simulink model "PID_mass_spring_damper_system"  (R2024a)
settings: Solver=ode3  StartTime=0.0  StopTime=inf  FixedStep=0.02  RelTol=1e-3
values from neighbouring files (symbols this model uses):
  b = 2    [param.m]
  k = 0.2    [param.m]
  m = 5    [param.m]
undefined symbols (not defined in the file or in its folder): DiscIntNeverNeededParam
libraries: robotlib x3, slpidlib x1
settings Model: Creator=Aras Güngöre  LastModifiedBy=fp_jin
settings SolverCC: AlgebraicLoopSolver=TrustRegion
settings DebuggingCC: UnconnectedInputMsg=warning  UnconnectedOutputMsg=warning  UnconnectedLineMsg=warning
settings ModelReferenceCC: EnableRefExpFcnMdlSchedulingChecks=on
settings RTWCC: GPUComputeCapability=3.5  DLArmComputeVersion=19.05

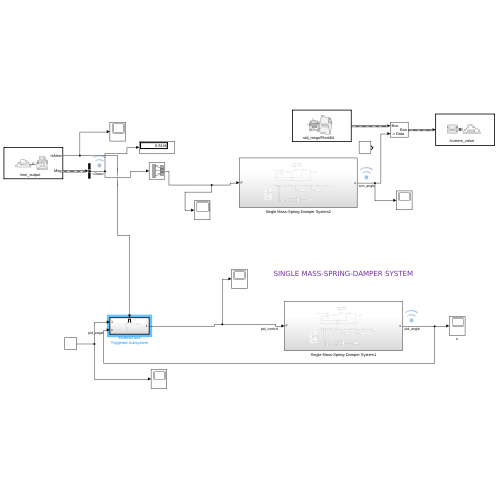
[thumbnail: Simulink's stored preview of the top-level diagram]
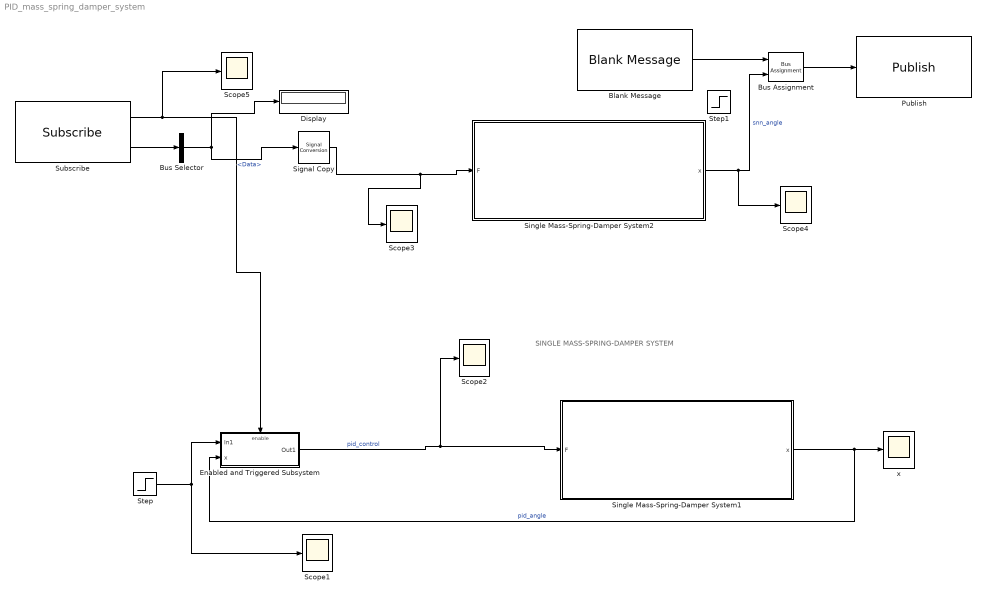
== system PID_mass_spring_damper_system ==
  note: SINGLE MASS-SPRING-DAMPER SYSTEM
  Blank Message : robotlib/Blank Message  messageClass=Message  entityType=std_msgs/Float64  messageType=std_msgs/Float64  SampleTime=-1  legacyBusStruct=off
  Bus Assignment : BusAssignment  AssignedSignals=Data
  Bus Selector : BusSelector  OutputSignals=Data
  Display : Display
  Enabled and Triggered Subsystem : Subsystem  TreatAsAtomicUnit=on
  Publish : robotlib/Publish  topicSource=Specify your own  topic=/current_value  messageType=std_msgs/Float64  legacyBusStruct=off  messageQueueLength=1
  Scope{1..5} (5 alike) : Scope
  Signal Copy : SignalConversion  OverrideOpt=off
  Single Mass-Spring-Damper System1 : Subsystem
  Single Mass-Spring-Damper System2 : Subsystem
  Step : Step  Time=0  After=5
  Step1 : Step  Time=0  After=15  SampleTime=0
  Subscribe : robotlib/Subscribe  topicSource=Specify your own  topic=/snn_output  messageType=std_msgs/Float64  SampleTime=-1  legacyBusStruct=off  messageQueueLength=1
  x : Scope
  wires:
  Blank Message/1 -> Bus Assignment/1
  Bus Assignment/1 -> Publish/1
  Bus Selector/1 -> Display/1, Signal Copy/1  "<Data>"
  Subscribe/2 -> Bus Selector/1
  Step/1 -> Enabled and Triggered Subsystem/1(In1), Scope1/1
  Enabled and Triggered Subsystem/1(Out1) -> Single Mass-Spring-Damper System1/1(F), Scope2/1  "pid_control"
  Single Mass-Spring-Damper System2/1(x) -> Bus Assignment/2, Scope4/1  "snn_angle"
  Signal Copy/1 -> Single Mass-Spring-Damper System2/1(F), Scope3/1
  Subscribe/1 -> Enabled and Triggered Subsystem/Enable, Scope5/1
  Single Mass-Spring-Damper System1/1(x) -> Enabled and Triggered Subsystem/2(x), x/1  "pid_angle"

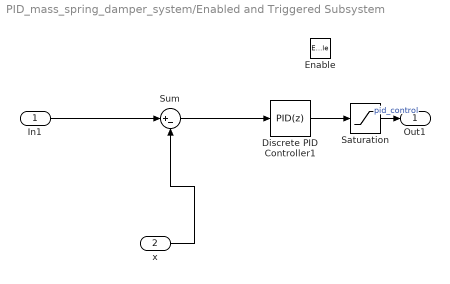
== system PID_mass_spring_damper_system/Enabled and Triggered Subsystem ==
  In1 : Inport
  x : Inport  Port=2
  Enable : EnablePort  StatesWhenEnabling=reset
  Discrete PID Controller1 : slpidlib/PID Controller  Controller=PID  Form=Parallel  TimeDomain=Discrete-time  UseExternalTs=off  SampleTime=-1  IntegratorMethod=Forward Euler  FilterMethod=Forward Euler  ControllerParametersSource=internal  P=1.72  I=0.238*1.0  UseKiTs=off  D=0.2*1.0  UseExternalDerivativeSource=off  N=100  UseFilter=off  TunerSelectOption=Transfer Function Based (PID Tuner App)  InitialConditionSource=internal  InitialConditionForIntegrator=0  InitialConditionForFilter=0  DifferentiatorICPrevScaledInput=0  ExternalReset=none  TrackingMode=off  Kt=1  LimitOutput=off  SatLimitsSource=internal  UpperSaturationLimit=inf  LowerSaturationLimit=-inf  LinearizeAsGain=off  AntiWindupMode=none  Kb=1  LimitIntegrator=off  UpperIntegratorSaturationLimit=inf  LowerIntegratorSaturationLimit=-inf  POutMin=[]  POutMax=[]  IOutMin=[]  IOutMax=[]  DOutMin=[]  DOutMax=[]  NOutMin=[]  NOutMax=[]  SumOutMin=[]  SumOutMax=[]  SaturationOutMin=[]  SaturationOutMax=[]  PParamMin=[]  PParamMax=[]  IParamMin=[]  IParamMax=[]  DParamMin=[]  DParamMax=[]  NParamMin=[]  NParamMax=[]  KbParamMin=[]  KbParamMax=[]  KtParamMin=[]  KtParamMax=[]  KbOutMin=[]  KbOutMax=[]  KtOutMin=[]  KtOutMax=[]  IntegratorOutMin=[]  IntegratorOutMax=[]  FilterOutMin=[]  FilterOutMax=[]  SumI1OutMin=[]  SumI1OutMax=[]  SumI2OutMin=[]  SumI2OutMax=[]  SumI3OutMin=[]  SumI3OutMax=[]  SumI4OutMin=[]  SumI4OutMax=[]  SumDOutMin=[]  SumDOutMax=[]  DifferentiatorOutMin=[]  DifferentiatorOutMax=[]  FilterDiffOutCoefMin=[]  FilterDiffOutCoefMax=[]  ReciprocalOutMin=[]  ReciprocalOutMax=[]  SumDenOutMin=[]  SumDenOutMax=[]  SumNumOutMin=[]  SumNumOutMax=[]  DivideOutMin=[]  DivideOutMax=[]  UdiffTsProdOutMin=[]  UdiffTsProdOutMax=[]  NTsProdOutMin=[]  NTsProdOutMax=[]  UintegralTsProdOutMin=[]  UintegralTsProdOutMax=[]  UngainTsProdOutMin=[]  UngainTsProdOutMax=[]  ClampingZeroOutDataTypeStr=Inherit: Inherit via back propagation  ClampingZeroOutMin=[]  ClampingZeroOutMax=[]  FilterDenConstantOutDataTypeStr=Inherit: Inherit via back propagation  FilterDenConstantOutMin=[]  FilterDenConstantOutMax=[]  PCopyOutDataTypeStr=Inherit: Inherit via back propagation  PCopyOutMin=[]  PCopyOutMax=[]  NCopyOutDataTypeStr=Inherit: Inherit via back propagation  NCopyOutMin=[]  NCopyOutMax=[]  IntegratorContinuousStateAttributes=''  IntegratorStateMustResolveToSignalObject=off  IntegratorRTWStateStorageClass=Auto  FilterContinuousStateAttributes=''  FilterStateMustResolveToSignalObject=off  FilterRTWStateStorageClass=Auto  ParallelPVariant=InternalParameters  IdealPVariant=Disabled  IVariant=InternalParameters  DVariant=InternalParameters  IntegratorVariant=Discrete  SatVariant=Disabled  AWVariant=Passthrough  PCopyVariant=Disabled  TRVariant=Disabled  FdbkBlocksVariant=Forward  IdealPFdbkVariant=Disabled  SatFdbkVariant=Disabled  DerivativeFilterVariant=Differentiator  NVariant=Passthrough  NCopyVariant=Disabled_SignalSpec  FilterICVariant=InternalICsDifferentiator  IntegratorICVariant=InternalICs  ExternalResetVariant=Disabled  TRSumVariant=Passthrough  SumFdbkVariant=Disabled  SumVariant=Sum_PID  TsampFilterVariant=InternalTs  TsampNgainVariant=Passthrough  TsampIntegralVariant=Disabled_SignalSpec  ExternalSaturationOutDataTypeStr=Inherit: Same as second input  DerivativeSourceVariant=ErrorSignal
      settings: LibrarySourceBlock=simulink/Discrete/Discrete PID Controller
  Saturation : Saturate  UpperLimit=20  LowerLimit=-20  LinearizeAsGain=off
  Sum : Sum  Inputs=|+-
  Out1 : Outport
  wires:
  In1/1 -> Sum/1
  Sum/1 -> Discrete PID Controller1/1
  x/1 -> Sum/2
  Discrete PID Controller1/1 -> Saturation/1
  Saturation/1 -> Out1/1  "pid_control"

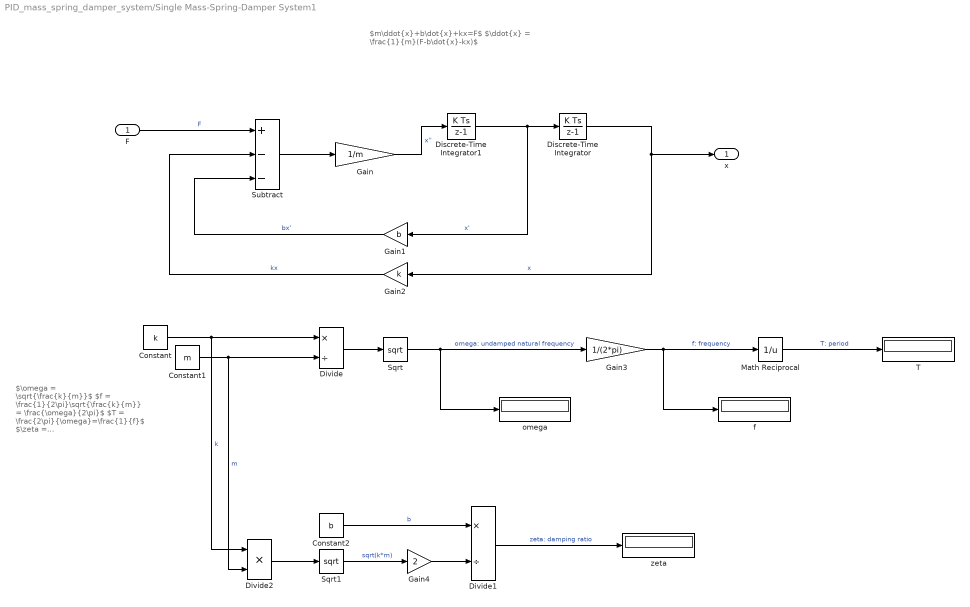
== system PID_mass_spring_damper_system/Single Mass-Spring-Damper System1 ==
  note: $\omega = \sqrt{\frac{k}{m}}$
      | $f = \frac{1}{2\pi}\sqrt{\frac{k}{m}} = \frac{\omega}{2\pi}$
      | $T = \frac{2\pi}{\omega}=\frac{1}{f}$
      | $\zeta = \frac{b}{2\sqrt{km}}$
  note: $m\ddot{x}+b\dot{x}+kx=F$
      | $\ddot{x} = \frac{1}{m}(F-b\dot{x}-kx)$
  F : Inport
  Constant : Constant  Value=k
  Constant1 : Constant  Value=m
  Constant2 : Constant  Value=b
  Discrete-Time Integrator : DiscreteIntegrator  SampleTime=-1  ICPrevOutput=DiscIntNeverNeededParam  ICPrevScaledInput=DiscIntNeverNeededParam
  Discrete-Time Integrator1 : DiscreteIntegrator  SampleTime=-1  ICPrevOutput=DiscIntNeverNeededParam  ICPrevScaledInput=DiscIntNeverNeededParam
  Divide : Product  Inputs=*/
  Divide1 : Product  Inputs=*/
  Divide2 : Product  Inputs=**
  Gain : Gain  Gain=1/m
  Gain1 : Gain  Gain=b
  Gain2 : Gain  Gain=k
  Gain3 : Gain  Gain=1/(2*pi)
  Gain4 : Gain  Gain=2
  Math Reciprocal : Math  Operator=reciprocal  SignedPower=on
  Sqrt : Sqrt
  Sqrt1 : Sqrt
  Subtract : Sum  Inputs=+--
  T : Display
  f : Display
  omega : Display
  zeta : Display
  x : Outport
  wires:
  Gain2/1 -> Subtract/2  "kx"
  Discrete-Time Integrator/1 -> x/1, Gain2/1  "x"
  F/1 -> Subtract/1  "F"
  Gain1/1 -> Subtract/3  "bx'"
  Discrete-Time Integrator1/1 -> Gain1/1, Discrete-Time Integrator/1  "x'"
  Subtract/1 -> Gain/1
  Gain/1 -> Discrete-Time Integrator1/1  "x''"
  Constant/1 -> Divide/1, Divide2/1  "k"
  Constant1/1 -> Divide2/2, Divide/2  "m"
  Divide/1 -> Sqrt/1
  Sqrt/1 -> omega/1, Gain3/1  "omega: undamped natural frequency"
  Gain3/1 -> f/1, Math Reciprocal/1  "f: frequency"
  Math Reciprocal/1 -> T/1  "T: period"
  Constant2/1 -> Divide1/1  "b"
  Sqrt1/1 -> Gain4/1  "sqrt(k*m)"
  Divide2/1 -> Sqrt1/1
  Divide1/1 -> zeta/1  "zeta: damping ratio"
  Gain4/1 -> Divide1/2

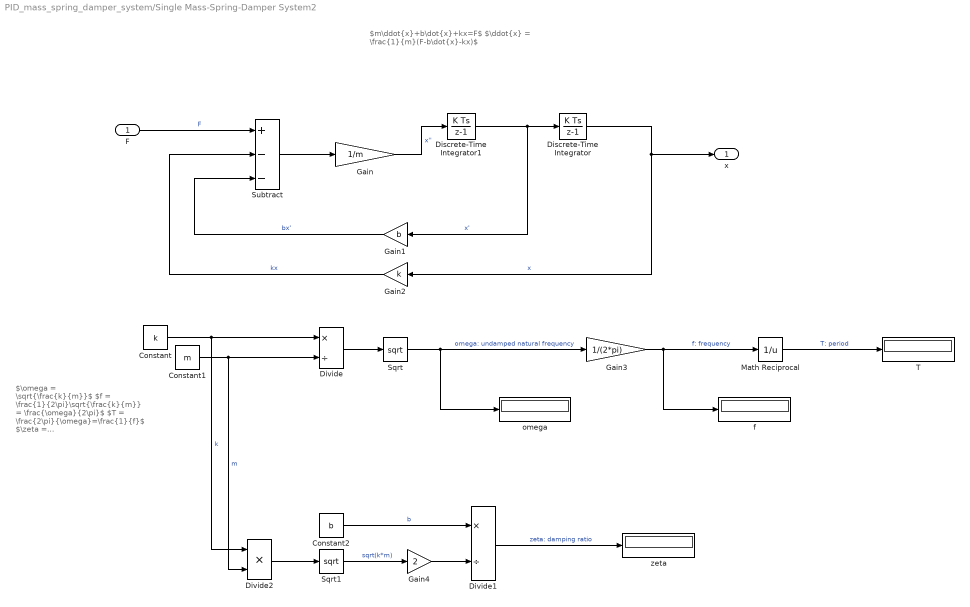
== system PID_mass_spring_damper_system/Single Mass-Spring-Damper System2 ==
  note: $\omega = \sqrt{\frac{k}{m}}$
      | $f = \frac{1}{2\pi}\sqrt{\frac{k}{m}} = \frac{\omega}{2\pi}$
      | $T = \frac{2\pi}{\omega}=\frac{1}{f}$
      | $\zeta = \frac{b}{2\sqrt{km}}$
  note: $m\ddot{x}+b\dot{x}+kx=F$
      | $\ddot{x} = \frac{1}{m}(F-b\dot{x}-kx)$
  F : Inport
  Constant : Constant  Value=k
  Constant1 : Constant  Value=m
  Constant2 : Constant  Value=b
  Discrete-Time Integrator : DiscreteIntegrator  SampleTime=-1  ICPrevOutput=DiscIntNeverNeededParam  ICPrevScaledInput=DiscIntNeverNeededParam
  Discrete-Time Integrator1 : DiscreteIntegrator  SampleTime=-1  ICPrevOutput=DiscIntNeverNeededParam  ICPrevScaledInput=DiscIntNeverNeededParam
  Divide : Product  Inputs=*/
  Divide1 : Product  Inputs=*/
  Divide2 : Product  Inputs=**
  Gain : Gain  Gain=1/m
  Gain1 : Gain  Gain=b
  Gain2 : Gain  Gain=k
  Gain3 : Gain  Gain=1/(2*pi)
  Gain4 : Gain  Gain=2
  Math Reciprocal : Math  Operator=reciprocal  SignedPower=on
  Sqrt : Sqrt
  Sqrt1 : Sqrt
  Subtract : Sum  Inputs=+--
  T : Display
  f : Display
  omega : Display
  zeta : Display
  x : Outport
  wires:
  Gain2/1 -> Subtract/2  "kx"
  Discrete-Time Integrator/1 -> x/1, Gain2/1  "x"
  F/1 -> Subtract/1  "F"
  Gain1/1 -> Subtract/3  "bx'"
  Discrete-Time Integrator1/1 -> Gain1/1, Discrete-Time Integrator/1  "x'"
  Subtract/1 -> Gain/1
  Gain/1 -> Discrete-Time Integrator1/1  "x''"
  Constant/1 -> Divide/1, Divide2/1  "k"
  Constant1/1 -> Divide2/2, Divide/2  "m"
  Divide/1 -> Sqrt/1
  Sqrt/1 -> omega/1, Gain3/1  "omega: undamped natural frequency"
  Gain3/1 -> f/1, Math Reciprocal/1  "f: frequency"
  Math Reciprocal/1 -> T/1  "T: period"
  Constant2/1 -> Divide1/1  "b"
  Sqrt1/1 -> Gain4/1  "sqrt(k*m)"
  Divide2/1 -> Sqrt1/1
  Divide1/1 -> zeta/1  "zeta: damping ratio"
  Gain4/1 -> Divide1/2
